simulink model "invertedPendulumModel"  (R2020b)
settings: Solver=VariableStepAuto  StartTime=0.0  StopTime=100  RelTol=1e-3
values from neighbouring files (symbols this model uses):
  A11 = Ab(1:2,1:2)    [TestesMalucos.m]
  A12 = Ab(1:2,3:4)    [TestesMalucos.m]
  A21 = Ab(3:4,1:2)    [TestesMalucos.m]
  A22 = Ab(3:4,3:4)    [TestesMalucos.m]
  b = 0.005    [TestesMalucos.m]
  B1 = Bb(1:2,:)    [TestesMalucos.m]
  B2 = Bb(3:4,:)    [TestesMalucos.m]
  ell = 2    [TestesMalucos.m]
  g = 9.8    [TestesMalucos.m]
  I = (m*ell^2)/3    (= 2.66666666667)    [TestesMalucos.m]
  Lb = L(3:4, :)    [TestesMalucos.m]
  m = 2    [TestesMalucos.m]
  M = 10    [TestesMalucos.m]
  Y1 = Y(:,1:2)    [TestesMalucos.m]
  Y2 = Y(:,3:4)    [TestesMalucos.m]
settings Model: Creator=lucianofrezzatto  LastModifiedBy=pedro
settings DebuggingCC: AlgebraicLoopMsg=none

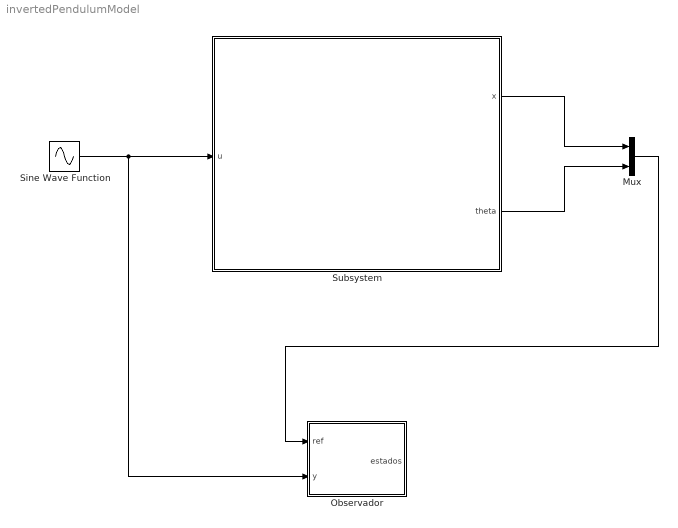
== system invertedPendulumModel ==
  Mux : Mux  Inputs=2
  Observador : Subsystem
  Sine Wave Function : Sin  SampleTime=0
  Subsystem : Subsystem  mask{m=m, Mc=M, I=I, l=ell, b=b, g=g, x0=0, dx0=0, th0=0, dth0=0}
      mask prompts: m "Massa do pêndulo (m)"; Mc "Massa do carro (M)"; I "Momento de inércia do pêndulo (I)"; l "Comprimento da haste (ell)"; b "Coeficiente de atrito viscoso"; g "Gravidade"; x0 "Posição inicial"; dx0 "Velocidade inicial"; th0 "Ângulo  inicial"; dth0 "Velocidade angular inicial"
      mask Display:
      | image('./invPend.png'); % Use "Edit Image" on toolstrip to change.
      | port_label('input',1,'u','texmode','on');
      | port_label('output',1,'x','texmode','on');
      | port_label('output',2,'\theta','texmode','on');
  wires:
  Sine Wave Function/1 -> Observador/2(y), Subsystem/1(u)
  Subsystem/1(x) -> Mux/1
  Subsystem/2(theta) -> Mux/2
  Mux/1 -> Observador/1(ref)

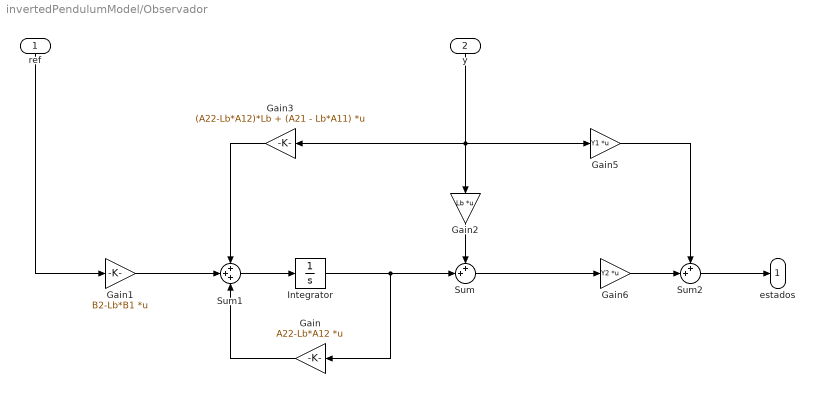
== system invertedPendulumModel/Observador ==
  ref : Inport
  y : Inport  Port=2
  Gain : Gain  Gain=A22-Lb*A12  Multiplication=Matrix(K*u) (u vector)
  Gain1 : Gain  Gain=B2-Lb*B1  Multiplication=Matrix(K*u) (u vector)
  Gain2 : Gain  Gain=Lb  Multiplication=Matrix(K*u) (u vector)
  Gain3 : Gain  Gain=(A22-Lb*A12)*Lb + (A21 - Lb*A11)  Multiplication=Matrix(K*u) (u vector)
  Gain5 : Gain  Gain=Y1  Multiplication=Matrix(K*u) (u vector)
  Gain6 : Gain  Gain=Y2  Multiplication=Matrix(K*u) (u vector)
  Integrator : Integrator
  Sum : Sum  Inputs=++|
  Sum1 : Sum  Inputs=+++
  Sum2 : Sum  Inputs=++|
  "estados " : Outport
  wires:
  Sum1/1 -> Integrator/1
  Integrator/1 -> Sum/2, Gain/1
  Gain/1 -> Sum1/3
  ref/1 -> Gain1/1
  Gain1/1 -> Sum1/2
  Gain3/1 -> Sum1/1
  y/1 -> Gain5/1, Gain3/1, Gain2/1
  Gain2/1 -> Sum/1
  Sum/1 -> Gain6/1
  Gain6/1 -> Sum2/2
  Sum2/1 -> "estados "/1
  Gain5/1 -> Sum2/1

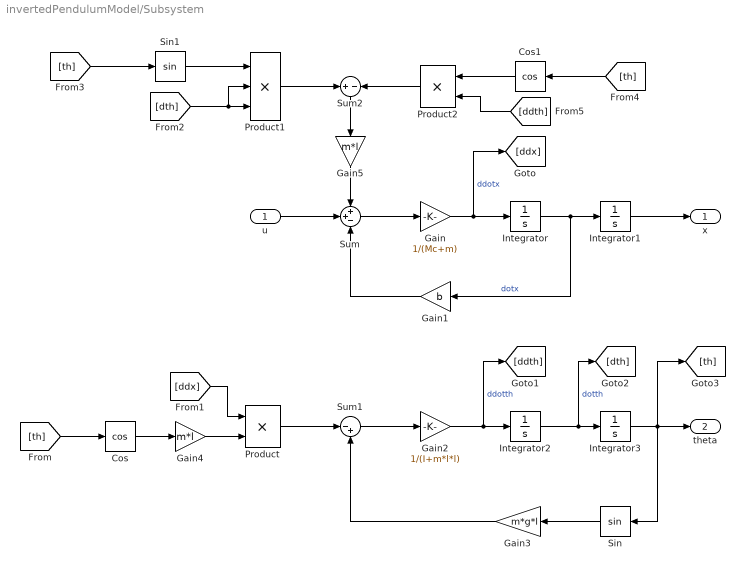
== system invertedPendulumModel/Subsystem ==
  u : Inport
  Cos : Trigonometry  Operator=cos
  Cos1 : Trigonometry  Operator=cos
  Gain : Gain  Gain=1/(Mc+m)
  Gain1 : Gain  Gain=b
  Gain2 : Gain  Gain=1/(I+m*l*l)
  Gain3 : Gain  Gain=m*g*l
  Gain4 : Gain  Gain=m*l
  Gain5 : Gain  Gain=m*l
  Integrator : Integrator  InitialCondition=dx0
  Integrator1 : Integrator  InitialCondition=x0
  Integrator2 : Integrator  InitialCondition=dth0
  Integrator3 : Integrator  InitialCondition=th0
  Product : Product
  Product1 : Product  Inputs=3
  Product2 : Product
  Sin : Trigonometry
  Sin1 : Trigonometry
  Sum : Sum  Inputs=++-
  Sum1 : Sum  Inputs=|-+
  Sum2 : Sum  Inputs=+-
  x : Outport
  theta : Outport  Port=2
  wires:
  Integrator/1 -> Integrator1/1, Gain1/1  "dotx"
  Integrator2/1 -> [dth], Integrator3/1  "dotth"
  Sum/1 -> Gain/1
  Gain/1 -> [ddx], Integrator/1  "ddotx"
  u/1 -> Sum/2
  Gain1/1 -> Sum/3
  Integrator1/1 -> x/1
  Integrator3/1 -> Sin/1, [th], theta/1
  Sum1/1 -> Gain2/1
  Gain2/1 -> [ddth], Integrator2/1  "ddotth"
  Sin/1 -> Gain3/1
  Gain3/1 -> Sum1/2
  Product/1 -> Sum1/1
  Gain4/1 -> Product/2
  [th] -> Cos/1
  Cos/1 -> Gain4/1
  [ddx] -> Product/1
  Gain5/1 -> Sum/1
  Sum2/1 -> Gain5/1
  Product1/1 -> Sum2/1
  [dth] -> Product1/2, Product1/3
  Sin1/1 -> Product1/1
  [th] -> Sin1/1
  Product2/1 -> Sum2/2
  Cos1/1 -> Product2/1
  [th] -> Cos1/1
  [ddth] -> Product2/2
